simulink model "Target_Control_System"  (R2021b)
settings: Solver=FixedStepDiscrete  StartTime=0.0  StopTime=5  RelTol=1e-3
PreLoadFcn:
  | RTWConfigurationCB('preloadfcn', bdroot);
PostLoadFcn:
  | load('configuration/data_struct.mat');
  | load('configuration/fluxMaps_propMotor.mat');
  | load('configuration/parameterInit_PROP.mat');
  | load('configuration/parameterInit_PUMP.mat');
  | load('configuration/parameterInit_PITCH.mat');
  | load('configuration/parameterInit_TILT.mat');
  | %load('configuration/base_workspace_signal_definition.mat');
  | %load('resolvedatastores_to_baseworkspace_for_faster_simulation.mat');
model workspace (MAT data in the model file):
  SIMULATION_OPTIONS : Simulink.Parameter (value not decoded)
  TARGET_CODE_GEN : Simulink.Parameter (value not decoded)
  TCS_SAMPLE_FREQ_HZ : Simulink.Parameter (value not decoded)
symbols that are objects in the model workspace (value not decoded): TARGET_CODE_GEN, TCS_SAMPLE_FREQ_HZ
undefined symbols (not defined in the file): A_DQ_REF_LPF_INIT__PITCH, A_DQ_REF_LPF_INIT__PROP, A_DQ_REF_LPF_INIT__PUMP, A_DQ_REF_LPF_INIT__TILT, A_OBSERVER_CONFIDENCE_INIT__PITCH, A_OBSERVER_CONFIDENCE_INIT__PROP, A_OBSERVER_CONFIDENCE_INIT__PUMP, A_OBSERVER_CONFIDENCE_INIT__TILT, ACTUATOR_MAX_ANGLE_TRIP__PITCH, ACTUATOR_MIN_ANGLE_TRIP__PITCH, ACTUATOR_POS_SENSOR_INV_DIRECTION__PITCH, ACTUATOR_POS_SENSOR_INV_DIRECTION__TILT, ACTUATOR_POS_SENSOR_OFFSET__PITCH, ACTUATOR_POS_SENSOR_OFFSET__TILT, ADC_scaler1_baseaddr_TILT, ADC_SCALER_FLOAT_TO_FIXPOINT_EXPANSION, ANGLE_ELEC_FROM_SENSOR_OFFSET_INIT__PITCH, ANGLE_ELEC_FROM_SENSOR_OFFSET_INIT__PROP, ANGLE_ELEC_FROM_SENSOR_OFFSET_INIT__PUMP, ANGLE_ELEC_FROM_SENSOR_OFFSET_INIT__TILT, AUTO_CLEAR_FAULTS_ENABLED__PITCH, AUTO_CLEAR_FAULTS_ENABLED__PROP, AUTO_CLEAR_FAULTS_ENABLED__PUMP, AUTO_CLEAR_FAULTS_ENABLED__TILT, AUTO_CLEAR_FAULTS_WAIT_TICKS__PITCH, AUTO_CLEAR_FAULTS_WAIT_TICKS__PROP, AUTO_CLEAR_FAULTS_WAIT_TICKS__PUMP, AUTO_CLEAR_FAULTS_WAIT_TICKS__TILT, AUTO_I_ZERO_IDLE_TICKS__PITCH, AUTO_I_ZERO_IDLE_TICKS__PROP, AUTO_I_ZERO_IDLE_TICKS__PUMP, AUTO_I_ZERO_IDLE_TICKS__TILT, AUTO_I_ZERO_OFFSET_IDC_THRESHOLD__PITCH, AUTO_I_ZERO_OFFSET_IDC_THRESHOLD__PROP, AUTO_I_ZERO_OFFSET_IDC_THRESHOLD__PUMP, AUTO_I_ZERO_OFFSET_IDC_THRESHOLD__TILT, AUTO_I_ZERO_OFFSET_IPH_THRESHOLD__PITCH, AUTO_I_ZERO_OFFSET_IPH_THRESHOLD__PROP, AUTO_I_ZERO_OFFSET_IPH_THRESHOLD__PUMP, AUTO_I_ZERO_OFFSET_IPH_THRESHOLD__TILT, AUTO_SENSORLESS_SWITCHOVER_DISABLE_OMEGA, AUTO_SENSORLESS_SWITCHOVER_ENABLE_OMEGA, AUTO_SENSORLESS_SWITCHOVER_MIN_CONFIDENCE, AUXILIARY_PROTECTION_UNIT_BASEADDR__TILT, blanking_max_error_omega_INIT_PITCH, blanking_max_error_omega_INIT_TILT, blanking_max_error_position_INIT_PITCH, blanking_max_error_position_INIT_TILT, BRUTE_START_I_Q_REF_RAMP_SPEED__PITCH, BRUTE_START_I_Q_REF_RAMP_SPEED__PROP, BRUTE_START_I_Q_REF_RAMP_SPEED__PUMP, BRUTE_START_I_Q_REF_RAMP_SPEED__TILT, CONTROL_LOOP_DT_INIT__PITCH, CONTROL_LOOP_DT_INIT__PROP, CONTROL_LOOP_DT_INIT__PUMP, CONTROL_LOOP_DT_INIT__TILT, CORRECTION_FILTER_SCALE__PITCH, CORRECTION_FILTER_SCALE__PROP, CORRECTION_FILTER_SCALE__PUMP, CORRECTION_FILTER_SCALE__TILT ... (+458)
libraries: simulink x178, Reusables_Lib x24
(part 5 of 47)

== system Target_Control_System/Target_Control_System/Simulation Controls/Simulation Data Store Initialization ==
  note: This function initializes all of the data store variables for simulation purposes. This mimics the parameter_init_prop.c and parameter_init_prop.h that are used for hardware execution.
      | If a variable is defined in parameter_init_prop.h, then it is included in the Model Workspace as a Simulink parameter.
  Constant76 : Constant  Value=0  SampleTime=-1
  Digital Clock : DigitalClock  SampleTime=-1
  Equal : RelationalOperator  Operator===  OutDataTypeStr=boolean  RndMeth=Simplest
  Function-Call Split{,1..6,8..9,17..27} (20 alike) : FunctionCallSplit  NumOutputPorts=2
  initializationFlowControl : Subsystem  TreatAsAtomicUnit=on
  initializeDataForPitch() : Subsystem  Priority=1  TreatAsAtomicUnit=on
  initializeDataForTilt() : Subsystem  Priority=1  TreatAsAtomicUnit=on
  initializeTiltAsMaster() : Subsystem
  parameter_init_prop : Subsystem  TreatAsAtomicUnit=on
  parameter_init_pump : Subsystem  TreatAsAtomicUnit=on
  setHardwareCurrentLimitTilt()1 : Subsystem  Commented=on  TreatAsAtomicUnit=on
  setPositionControlModeTilt() : Subsystem
  setTiltMotorSpecificParameters() : Subsystem
  setupIirFilters(&oTilt) : Subsystem
  setupIirFilters() : Subsystem
  setupObserver(&oTilt) : Subsystem  TreatAsAtomicUnit=on
  setupObserver() : Subsystem
  setupObserverForPosSensor(&oTilt) : Subsystem
  setupPwm(&oTilt) : Subsystem
  setupPwm() : Subsystem
  updateIqSetpointMax(&oTilt) : Subsystem
  updateIqSetpointMax() : Subsystem
  updateServoObserver(&oTilt) : Subsystem
  updateServoObserver() : Subsystem
  updateSoftCurrentLimitTilt()1 : Subsystem  Commented=on  TreatAsAtomicUnit=on
  wires:
  Function-Call Split21/2 -> Function-Call Split20/1
  Function-Call Split9/1 -> updateIqSetpointMax()/Trigger
  Function-Call Split27/2 -> Function-Call Split19/1
  Function-Call Split22/1 -> updateIqSetpointMax(&oTilt)/Trigger
  Function-Call Split23/1 -> initializeTiltAsMaster()/Trigger
  Function-Call Split20/2 -> updateSoftCurrentLimitTilt()1/Trigger
  Function-Call Split24/2 -> Function-Call Split25/1
  Function-Call Split26/1 -> updateServoObserver(&oTilt)/Trigger
  Function-Call Split23/2 -> Function-Call Split21/1
  Function-Call Split18/2 -> Function-Call Split24/1
  Function-Call Split24/1 -> setupPwm(&oTilt)/Trigger
  Function-Call Split2/2 -> Function-Call Split17/1
  Function-Call Split19/2 -> Function-Call Split22/1
  Function-Call Split21/1 -> setPositionControlModeTilt()/Trigger
  Function-Call Split17/1 -> initializeDataForTilt()/Trigger
  Function-Call Split17/2 -> Function-Call Split18/1
  Function-Call Split26/2 -> Function-Call Split27/1
  Function-Call Split25/1 -> setupObserver(&oTilt)/Trigger
  Function-Call Split18/1 -> setTiltMotorSpecificParameters()/Trigger
  Function-Call Split27/1 -> setupObserverForPosSensor(&oTilt)/Trigger
  Function-Call Split20/1 -> setHardwareCurrentLimitTilt()1/Trigger
  Function-Call Split25/2 -> Function-Call Split26/1
  Function-Call Split22/2 -> Function-Call Split23/1
  Function-Call Split19/1 -> setupIirFilters(&oTilt)/Trigger
  Function-Call Split1/1 -> parameter_init_pump/Trigger
  Function-Call Split5/1 -> updateServoObserver()/Trigger
  Function-Call Split3/1 -> setupPwm()/Trigger
  Function-Call Split6/1 -> setupIirFilters()/Trigger
  Function-Call Split4/2 -> Function-Call Split5/1
  Function-Call Split4/1 -> setupObserver()/Trigger
  Function-Call Split5/2 -> Function-Call Split6/1
  Function-Call Split8/2 -> Function-Call Split3/1
  Function-Call Split6/2 -> Function-Call Split9/1
  Function-Call Split8/1 -> initializeDataForPitch()/Trigger
  Function-Call Split3/2 -> Function-Call Split4/1
  Equal/1 -> initializationFlowControl/Trigger
  Function-Call Split1/2 -> Function-Call Split2/1
  initializationFlowControl/1(Out1) -> Function-Call Split/1
  Function-Call Split/1 -> parameter_init_prop/Trigger
  Function-Call Split/2 -> Function-Call Split1/1
  Function-Call Split2/1 -> Function-Call Split8/1
  Constant76/1 -> Equal/2
  Digital Clock/1 -> Equal/1

== system Target_Control_System/Target_Control_System/Simulation Controls/pitchMotor ==
  pitchMotor_simControls : Inport
  Apply Simulation Parameter Values : Subsystem  TreatAsAtomicUnit=on
  Apply Simulation Setpoints : Subsystem  TreatAsAtomicUnit=on
  Bus Selector : BusSelector  OutputSignals=uiEnable
  Bus Selector1 : BusSelector  OutputSignals=controlSelector
  Bus Selector2 : BusSelector  OutputSignals=currentSetpoint,speedSetpoint,positionSetpoint
  Bus Selector3 : BusSelector  OutputSignals=OneOverSensorPolePairs
  Detect Change : simulink/Logic and Bit Operations/Detect Change  vinit=0  OutDataTypeStr=boolean
  Detect Change1 : simulink/Logic and Bit Operations/Detect Change  vinit=0  OutDataTypeStr=boolean
  Drive Enable : Subsystem  TreatAsAtomicUnit=on
  Initialize controller : Subsystem  TreatAsAtomicUnit=on
  wires:
  Bus Selector2/3 -> Apply Simulation Setpoints/4(Position Setpoint for Simulation)  "<positionSetpoint>"
  Bus Selector2/1 -> Apply Simulation Setpoints/2(Current Setpoint for Simulation)  "<currentSetpoint>"
  Bus Selector2/2 -> Apply Simulation Setpoints/3(Speed Setpoint for Simulation)  "<speedSetpoint>"
  Bus Selector1/1 -> Initialize controller/1(controllerSelection), Apply Simulation Setpoints/1(controllerSelection), Detect Change1/1  "<controlSelector>"
  pitchMotor_simControls/1 -> Bus Selector/1, Bus Selector3/1, Bus Selector2/1, Bus Selector1/1
  Detect Change1/1 -> Initialize controller/Trigger  "change"
  Bus Selector3/1 -> Apply Simulation Parameter Values/1(OneOverSensorPolePairs)  "<OneOverSensorPolePairs>"
  Bus Selector/1 -> Detect Change/1, Drive Enable/1(pitchMotor_uiEnable)  "<uiEnable>"
  Detect Change/1 -> Drive Enable/Trigger  "change"

== system Target_Control_System/Target_Control_System/Simulation Controls/pitchMotor1 ==
  pitchMotor_fpgaFeedback : Inport
  Bus Selector : BusSelector  OutputSignals=oPitch:oMot_:oOut_:uiGateDriverStatus_,mdl_pitch_uiFlags,mdl_pitch_uiAPUFlags,oPitch:oMot_:oState_:opInputResolverData_:uiControlReadback_
  Data Store Write : DataStoreWrite  DataStoreName=oPitch  DataStoreElements=oPitch.oMot_.oState_.opInputResolverData_.uiControlReadback_  IndexOptions=Index vector (dialog)  Indices=1  OutputSizes=1
  Data Store Write1 : DataStoreWrite  DataStoreName=mdl_pitch_uiFlags  IndexOptions=Index vector (dialog)  Indices=1  OutputSizes=1
  Data Store Write2 : DataStoreWrite  DataStoreName=mdl_pitch_uiAPUFlags  IndexOptions=Index vector (dialog)  Indices=1  OutputSizes=1
  Data Store Write43 : DataStoreWrite  DataStoreName=oPitch  DataStoreElements=oPitch.oMot_.oOut_.uiGateDriverStatus_  IndexOptions=Index vector (dialog)  Indices=1  OutputSizes=1
  wires:
  Bus Selector/4 -> Data Store Write/1  "<oPitch:oMot_:oState_:opInputResolverData_:uiControlReadback_>"
  pitchMotor_fpgaFeedback/1 -> Bus Selector/1
  Bus Selector/2 -> Data Store Write1/1  "<mdl_pitch_uiFlags>"
  Bus Selector/3 -> Data Store Write2/1  "<mdl_pitch_uiAPUFlags>"
  Bus Selector/1 -> Data Store Write43/1  "<oPitch:oMot_:oOut_:uiGateDriverStatus_>"

== system Target_Control_System/Target_Control_System/Simulation Controls/propMotor ==
  propMotor_simControls : Inport
  Bus Selector : BusSelector  OutputSignals=uiEnable
  Detect Change : simulink/Logic and Bit Operations/Detect Change  vinit=0  OutDataTypeStr=boolean
  Drive Enable : Subsystem  TreatAsAtomicUnit=on
  wires:
  Bus Selector/1 -> Drive Enable/1(propMotor_uiEnable), Detect Change/1  "<uiEnable>"
  propMotor_simControls/1 -> Bus Selector/1
  Detect Change/1 -> Drive Enable/Trigger  "change"

== system Target_Control_System/Target_Control_System/Simulation Controls/pumpMotor ==
  pitchMotor_simControls : Inport
  Bus Selector : BusSelector  OutputSignals=uiEnable
  Detect Change : simulink/Logic and Bit Operations/Detect Change  vinit=0  OutDataTypeStr=boolean
  Drive Enable : Subsystem  TreatAsAtomicUnit=on
  wires:
  Bus Selector/1 -> Drive Enable/1(pumpMotor_uiEnable), Detect Change/1  "<uiEnable>"
  pitchMotor_simControls/1 -> Bus Selector/1  "pumpMotor_simControls"
  Detect Change/1 -> Drive Enable/Trigger  "change"

== system Target_Control_System/Target_Control_System/Simulation Controls/tiltMotor ==
  pitchMotor_simControls : Inport
  Apply Simulation Parameter Values : Subsystem  TreatAsAtomicUnit=on
  Apply Simulation Setpoints : Subsystem  TreatAsAtomicUnit=on
  Bus Selector : BusSelector  OutputSignals=uiEnable
  Bus Selector1 : BusSelector  OutputSignals=controlSelector
  Bus Selector2 : BusSelector  OutputSignals=currentSetpoint,speedSetpoint,positionSetpoint
  Bus Selector3 : BusSelector  OutputSignals=OneOverSensorPolePairs,TiltReadheadCompensationEnabled
  Detect Change : simulink/Logic and Bit Operations/Detect Change  vinit=0  OutDataTypeStr=boolean
  Detect Change1 : simulink/Logic and Bit Operations/Detect Change  vinit=0  OutDataTypeStr=boolean
  Drive Enable : Subsystem  TreatAsAtomicUnit=on
  Initialize controller : Subsystem  TreatAsAtomicUnit=on
  wires:
  Detect Change1/1 -> Initialize controller/Trigger  "change"
  Bus Selector2/2 -> Apply Simulation Setpoints/3(Speed Setpoint for Simulation)  "<speedSetpoint>"
  Bus Selector2/1 -> Apply Simulation Setpoints/2(Current Setpoint for Simulation)  "<currentSetpoint>"
  Bus Selector2/3 -> Apply Simulation Setpoints/4(Position Setpoint for Simulation)  "<positionSetpoint>"
  Bus Selector1/1 -> Initialize controller/1(controllerSelection), Apply Simulation Setpoints/1(controllerSelection), Detect Change1/1  "<controlSelector>"
  Bus Selector3/2 -> Apply Simulation Parameter Values/2(TiltReadheadCompensationEnabled)  "<TiltReadheadCompensationEnabled>"
  Bus Selector3/1 -> Apply Simulation Parameter Values/1(OneOverSensorPolePairs)  "<OneOverSensorPolePairs>"
  Bus Selector/1 -> Drive Enable/1(tiltMotor_uiEnable), Detect Change/1  "<uiEnable>"
  pitchMotor_simControls/1 -> Bus Selector/1, Bus Selector3/1, Bus Selector2/1, Bus Selector1/1  "tiltMotor_simControls"
  Detect Change/1 -> Drive Enable/Trigger  "change"

== system Target_Control_System/Target_Control_System/Simulation Controls/tiltMotor1 ==
  tiltMotor_fpgaFeedback : Inport
  Bus Selector : BusSelector  OutputSignals=oTilt:oMot_:oOut_:uiGateDriverStatus_,mdl_tilt_uiFlags,mdl_tilt_uiAPUFlags,oTilt:oMot_:oState_:opInputResolverData_:uiControlReadback_,mdl_tilt_uiInputSensorFlags,mdl_tilt_uiOutputSensorFlags
  Data Store Write : DataStoreWrite  DataStoreName=oTilt  DataStoreElements=oTilt.oMot_.oState_.opInputResolverData_.uiControlReadback_  IndexOptions=Index vector (dialog)  Indices=1  OutputSizes=1
  Data Store Write1 : DataStoreWrite  DataStoreName=mdl_tilt_uiFlags  IndexOptions=Index vector (dialog)  Indices=1  OutputSizes=1
  Data Store Write2 : DataStoreWrite  DataStoreName=mdl_tilt_uiAPUFlags  IndexOptions=Index vector (dialog)  Indices=1  OutputSizes=1
  Data Store Write3 : DataStoreWrite  DataStoreName=mdl_tilt_uiInputSensorFlags  IndexOptions=Index vector (dialog)  Indices=1  OutputSizes=1
  Data Store Write4 : DataStoreWrite  DataStoreName=mdl_tilt_uiOutputSensorFlags  IndexOptions=Index vector (dialog)  Indices=1  OutputSizes=1
  Data Store Write43 : DataStoreWrite  DataStoreName=oTilt  DataStoreElements=oTilt.oMot_.oOut_.uiGateDriverStatus_  IndexOptions=Index vector (dialog)  Indices=1  OutputSizes=1
  wires:
  Bus Selector/6 -> Data Store Write4/1  "<mdl_tilt_uiOutputSensorFlags>"
  Bus Selector/5 -> Data Store Write3/1  "<mdl_tilt_uiInputSensorFlags>"
  Bus Selector/4 -> Data Store Write/1  "<oTilt:oMot_:oState_:opInputResolverData_:uiControlReadback_>"
  tiltMotor_fpgaFeedback/1 -> Bus Selector/1
  Bus Selector/2 -> Data Store Write1/1  "<mdl_tilt_uiFlags>"
  Bus Selector/3 -> Data Store Write2/1  "<mdl_tilt_uiAPUFlags>"
  Bus Selector/1 -> Data Store Write43/1  "<oTilt:oMot_:oOut_:uiGateDriverStatus_>"

== system Target_Control_System/Target_Control_System/DEBUG_Scopes/Pump Motor Debug/2Pi_Mod1 ==
  Iabc1 : Inport
  Constant : Constant  Value=pi  OutDataTypeStr=single  SampleTime=-1
  "Constant " : Constant  Value=pi  OutDataTypeStr=single  SampleTime=-1
  Math Function : Math  Operator=mod  SignedPower=on  SaturateOnIntegerOverflow=on
  Modulo Constant : Constant  Value=2*pi  OutDataTypeStr=single  SampleTime=-1
  Sum1 : Sum  Inputs=|++
  Sum2 : Sum  Inputs=|+-
  Out1 : Outport
  wires:
  Sum2/1 -> Out1/1
  Constant/1 -> Sum2/2
  Math Function/1 -> Sum2/1
  Sum1/1 -> Math Function/1
  Iabc1/1 -> Sum1/1
  "Constant "/1 -> Sum1/2
  Modulo Constant/1 -> Math Function/2

== system Target_Control_System/Target_Control_System/DEBUG_Scopes/Pump Motor Debug/2Pi_Mod2 ==
  Iabc1 : Inport
  Discrete Integrator Samples1 : Constant  Value=270/360*2*pi  OutDataTypeStr=single  SampleTime=-1
  Discrete Integrator Samples2 : Constant  Value=pi  OutDataTypeStr=single  SampleTime=-1
  Math Function : Math  Operator=mod  SignedPower=on  SaturateOnIntegerOverflow=on
  Modulo Constant : Constant  Value=2*pi  OutDataTypeStr=single  SampleTime=-1
  Sum1 : Sum  Inputs=|++
  Sum2 : Sum  Inputs=|+-
  Out1 : Outport
  wires:
  Sum2/1 -> Out1/1
  Discrete Integrator Samples2/1 -> Sum2/2
  Math Function/1 -> Sum2/1
  Sum1/1 -> Math Function/1
  Iabc1/1 -> Sum1/1
  Discrete Integrator Samples1/1 -> Sum1/2
  Modulo Constant/1 -> Math Function/2

== system Target_Control_System/Target_Control_System/DEBUG_Scopes/Pump Motor Debug/IIR3 ==
  Input : Inport
  Constant : Constant  Value=CoefficientA  OutDataTypeStr=single  SampleTime=-1
  Constant1 : Constant  Value=CoefficientB  OutDataTypeStr=single  SampleTime=-1
  Product : Product  OutDataTypeStr=single  RndMeth=Zero
  Product1 : Product  RndMeth=Zero
  Sum : Sum  Inputs=|++  OutDataTypeStr=single
  Unit Delay : UnitDelay  SampleTime=-1  HasFrameUpgradeWarning=on
  Output : Outport
  wires:
  Sum/1 -> Unit Delay/1, Output/1
  Unit Delay/1 -> Product/1
  Constant1/1 -> Product1/2
  Constant/1 -> Product/2
  Product/1 -> Sum/1
  Product1/1 -> Sum/2
  Input/1 -> Product1/1

== system Target_Control_System/Target_Control_System/DEBUG_Scopes/Pump Motor Debug/IIR4 ==
  Input : Inport
  Constant : Constant  Value=CoefficientA  OutDataTypeStr=single  SampleTime=-1
  Constant1 : Constant  Value=CoefficientB  OutDataTypeStr=single  SampleTime=-1
  Product : Product  OutDataTypeStr=single  RndMeth=Zero
  Product1 : Product  RndMeth=Zero
  Sum : Sum  Inputs=|++  OutDataTypeStr=single
  Unit Delay : UnitDelay  SampleTime=-1  HasFrameUpgradeWarning=on
  Output : Outport
  wires:
  Sum/1 -> Unit Delay/1, Output/1
  Unit Delay/1 -> Product/1
  Constant1/1 -> Product1/2
  Constant/1 -> Product/2
  Product/1 -> Sum/1
  Product1/1 -> Sum/2
  Input/1 -> Product1/1

== system Target_Control_System/Target_Control_System/InterruptFunction/allMotors_readAdc/codeGen_adcRead ==
  Enable : EnablePort
  Data Store Read24 : DataStoreRead  DataStoreName=oProp  DataStoreElements=oProp.oIsr_.oIn_.oAdcData_.fUa_  IndexOptions=Index vector (dialog)  Indices=1  OutputSizes=1
  Data Store Read25 : DataStoreRead  DataStoreName=oProp  DataStoreElements=oProp.oIsr_.oIn_.oAdcData_.fUb_  IndexOptions=Index vector (dialog)  Indices=1  OutputSizes=1
  Data Store Read26 : DataStoreRead  DataStoreName=oProp  DataStoreElements=oProp.oIsr_.oIn_.oAdcData_.fUc_  IndexOptions=Index vector (dialog)  Indices=1  OutputSizes=1
  Data Store Read27 : DataStoreRead  DataStoreName=oPitch  DataStoreElements=oPitch.oIsr_.oIn_.oAdcData_.fUa_  IndexOptions=Index vector (dialog)  Indices=1  OutputSizes=1
  Data Store Read30 : DataStoreRead  DataStoreName=oPitch  DataStoreElements=oPitch.oIsr_.oIn_.oAdcData_.fUb_  IndexOptions=Index vector (dialog)  Indices=1  OutputSizes=1
  Data Store Read33 : DataStoreRead  DataStoreName=oPump  DataStoreElements=oPump.oIsr_.oIn_.oAdcData_.fUa_  IndexOptions=Index vector (dialog)  Indices=1  OutputSizes=1
  Data Store Read34 : DataStoreRead  DataStoreName=oPump  DataStoreElements=oPump.oIsr_.oIn_.oAdcData_.fUb_  IndexOptions=Index vector (dialog)  Indices=1  OutputSizes=1
  Data Store Read35 : DataStoreRead  DataStoreName=oPump  DataStoreElements=oPump.oIsr_.oIn_.oAdcData_.fUc_  IndexOptions=Index vector (dialog)  Indices=1  OutputSizes=1
  Data Store Read36 : DataStoreRead  DataStoreName=oPitch  DataStoreElements=oPitch.oIsr_.oIn_.oAdcData_.fUc_  IndexOptions=Index vector (dialog)  Indices=1  OutputSizes=1
  Data Store Read39 : DataStoreRead  DataStoreName=oTilt  DataStoreElements=oTilt.oIsr_.oIn_.oAdcData_.fUa_  IndexOptions=Index vector (dialog)  Indices=1  OutputSizes=1
  Data Store Read4 : DataStoreRead  DataStoreName=oPump  DataStoreElements=oPump.oIsr_.oIn_.oAdcData_.fUdc_  IndexOptions=Index vector (dialog)  Indices=1  OutputSizes=1
  Data Store Read41 : DataStoreRead  DataStoreName=oTilt  DataStoreElements=oTilt.oIsr_.oIn_.oAdcData_.fUb_  IndexOptions=Index vector (dialog)  Indices=1  OutputSizes=1
  Data Store Read42 : DataStoreRead  DataStoreName=oTilt  DataStoreElements=oTilt.oIsr_.oIn_.oAdcData_.fUc_  IndexOptions=Index vector (dialog)  Indices=1  OutputSizes=1
  Data Store Read8 : DataStoreRead  DataStoreName=oProp  DataStoreElements=oProp.oIsr_.oIn_.oAdcData_.fUdc_  IndexOptions=Index vector (dialog)  Indices=1  OutputSizes=1
  Data Store Write10 : DataStoreWrite  DataStoreName=oTilt  DataStoreElements=oTilt.oIsr_.oState_.fUdcPostlpf_  IndexOptions=Index vector (dialog)  Indices=1  OutputSizes=1
  Data Store Write11 : DataStoreWrite  DataStoreName=oProp  DataStoreElements=oProp.oIsr_.oState_.fUaPostlpf_  IndexOptions=Index vector (dialog)  Indices=1  OutputSizes=1
  Data Store Write12 : DataStoreWrite  DataStoreName=oProp  DataStoreElements=oProp.oIsr_.oState_.fUbPostlpf_  IndexOptions=Index vector (dialog)  Indices=1  OutputSizes=1
  Data Store Write13 : DataStoreWrite  DataStoreName=oProp  DataStoreElements=oProp.oIsr_.oState_.fUcPostlpf_  IndexOptions=Index vector (dialog)  Indices=1  OutputSizes=1
  Data Store Write22 : DataStoreWrite  DataStoreName=oPump  DataStoreElements=oPump.oIsr_.oState_.fUaPostlpf_  IndexOptions=Index vector (dialog)  Indices=1  OutputSizes=1
  Data Store Write23 : DataStoreWrite  DataStoreName=oPump  DataStoreElements=oPump.oIsr_.oState_.fUbPostlpf_  IndexOptions=Index vector (dialog)  Indices=1  OutputSizes=1
  Data Store Write24 : DataStoreWrite  DataStoreName=oPump  DataStoreElements=oPump.oIsr_.oState_.fUcPostlpf_  IndexOptions=Index vector (dialog)  Indices=1  OutputSizes=1
  Data Store Write3 : DataStoreWrite  DataStoreName=oPitch  DataStoreElements=oPitch.oIsr_.oIn_.oAdcData_.fUdc_  IndexOptions=Index vector (dialog)  Indices=1  OutputSizes=1
  Data Store Write31 : DataStoreWrite  DataStoreName=oPitch  DataStoreElements=oPitch.oIsr_.oState_.fUaPostlpf_  IndexOptions=Index vector (dialog)  Indices=1  OutputSizes=1
  Data Store Write32 : DataStoreWrite  DataStoreName=oPitch  DataStoreElements=oPitch.oIsr_.oState_.fUbPostlpf_  IndexOptions=Index vector (dialog)  Indices=1  OutputSizes=1
  Data Store Write33 : DataStoreWrite  DataStoreName=oPitch  DataStoreElements=oPitch.oIsr_.oState_.fUcPostlpf_  IndexOptions=Index vector (dialog)  Indices=1  OutputSizes=1
  Data Store Write37 : DataStoreWrite  DataStoreName=oTilt  DataStoreElements=oTilt.oIsr_.oState_.fUaPostlpf_  IndexOptions=Index vector (dialog)  Indices=1  OutputSizes=1
  Data Store Write38 : DataStoreWrite  DataStoreName=oTilt  DataStoreElements=oTilt.oIsr_.oState_.fUbPostlpf_  IndexOptions=Index vector (dialog)  Indices=1  OutputSizes=1
  Data Store Write39 : DataStoreWrite  DataStoreName=oTilt  DataStoreElements=oTilt.oIsr_.oState_.fUcPostlpf_  IndexOptions=Index vector (dialog)  Indices=1  OutputSizes=1
  Data Store Write4 : DataStoreWrite  DataStoreName=oPump  DataStoreElements=oPump.oIsr_.oState_.fUdcPostlpf_  IndexOptions=Index vector (dialog)  Indices=1  OutputSizes=1
  Data Store Write5 : DataStoreWrite  DataStoreName=oProp  DataStoreElements=oProp.oIsr_.oState_.fUdcPostlpf_  IndexOptions=Index vector (dialog)  Indices=1  OutputSizes=1
  Data Store Write6 : DataStoreWrite  DataStoreName=oTilt  DataStoreElements=oTilt.oIsr_.oIn_.oAdcData_.fUdc_  IndexOptions=Index vector (dialog)  Indices=1  OutputSizes=1
  Data Store Write7 : DataStoreWrite  DataStoreName=oPitch  DataStoreElements=oPitch.oIsr_.oState_.fUdcPostlpf_  IndexOptions=Index vector (dialog)  Indices=1  OutputSizes=1
  wires:
  Data Store Read8/1 -> Data Store Write5/1  "Udc"
  Data Store Read4/1 -> Data Store Write4/1, Data Store Write3/1, Data Store Write7/1, Data Store Write6/1, Data Store Write10/1  "Ua"
  Data Store Read39/1 -> Data Store Write37/1
  Data Store Read41/1 -> Data Store Write38/1
  Data Store Read27/1 -> Data Store Write31/1
  Data Store Read25/1 -> Data Store Write12/1
  Data Store Read42/1 -> Data Store Write39/1
  Data Store Read24/1 -> Data Store Write11/1
  Data Store Read34/1 -> Data Store Write23/1
  Data Store Read30/1 -> Data Store Write32/1
  Data Store Read35/1 -> Data Store Write24/1
  Data Store Read33/1 -> Data Store Write22/1
  Data Store Read26/1 -> Data Store Write13/1
  Data Store Read36/1 -> Data Store Write33/1

== system Target_Control_System/Target_Control_System/InterruptFunction/allMotors_readAdc/pitchMotor_adcRead ==
  PitchMotorAdcFeedback : Inport  OutDataTypeStr=Bus: SAdcDataSingleIn_t  PortDimensions=[ 1 ]  BusOutputAsStruct=on
  Enable : EnablePort
  Bus Selector : BusSelector  OutputSignals=fIa_,fIb_,fIc_,fIdc_,fUa_,fUb_,fUc_,fUdc_,fAuxiliaryEncoderFloat_,fMotorEncoderFloat_,fMotorSensorSpeed_,fOutputEncoderFloat_,fOutputSensorSpeed_
  Data Store Write : DataStoreWrite  DataStoreName=oPitch  DataStoreElements=oPitch.oIsr_.oIn_.oAdcData_.fIa_  IndexOptions=Index vector (dialog)  Indices=1  OutputSizes=1
  Data Store Write1 : DataStoreWrite  DataStoreName=oPitch  DataStoreElements=oPitch.oIsr_.oIn_.oAdcData_.fIb_  IndexOptions=Index vector (dialog)  Indices=1  OutputSizes=1
  Data Store Write10 : DataStoreWrite  DataStoreName=oPitch  DataStoreElements=oPitch.oIsr_.oIn_.oAdcData_.fMotorSensorSpeed_  IndexOptions=Index vector (dialog)  Indices=1  OutputSizes=1
  Data Store Write11 : DataStoreWrite  DataStoreName=oPitch  DataStoreElements=oPitch.oIsr_.oIn_.oAdcData_.fOutputEncoderFloat_  IndexOptions=Index vector (dialog)  Indices=1  OutputSizes=1
  Data Store Write12 : DataStoreWrite  DataStoreName=oPitch  DataStoreElements=oPitch.oIsr_.oIn_.oAdcData_.fOutputSensorSpeed_  IndexOptions=Index vector (dialog)  Indices=1  OutputSizes=1
  Data Store Write13 : DataStoreWrite  DataStoreName=oPitch  DataStoreElements=oPitch.oIsr_.oOut_.fUdc_  IndexOptions=Index vector (dialog)  Indices=1  OutputSizes=1
  Data Store Write14 : DataStoreWrite  DataStoreName=oPitch  DataStoreElements=oPitch.oIsr_.oState_.fUaPostlpf_  IndexOptions=Index vector (dialog)  Indices=1  OutputSizes=1
  Data Store Write15 : DataStoreWrite  DataStoreName=oPitch  DataStoreElements=oPitch.oIsr_.oState_.fUbPostlpf_  IndexOptions=Index vector (dialog)  Indices=1  OutputSizes=1
  Data Store Write16 : DataStoreWrite  DataStoreName=oPitch  DataStoreElements=oPitch.oIsr_.oState_.fUcPostlpf_  IndexOptions=Index vector (dialog)  Indices=1  OutputSizes=1
  Data Store Write19 : DataStoreWrite  DataStoreName=oPitch  DataStoreElements=oPitch.oIsr_.oState_.fUdcPostlpf_  IndexOptions=Index vector (dialog)  Indices=1  OutputSizes=1
  Data Store Write2 : DataStoreWrite  DataStoreName=oPitch  DataStoreElements=oPitch.oIsr_.oIn_.oAdcData_.fIc_  IndexOptions=Index vector (dialog)  Indices=1  OutputSizes=1
  Data Store Write3 : DataStoreWrite  DataStoreName=oPitch  DataStoreElements=oPitch.oIsr_.oIn_.oAdcData_.fIdc_  IndexOptions=Index vector (dialog)  Indices=1  OutputSizes=1
  Data Store Write4 : DataStoreWrite  DataStoreName=oPitch  DataStoreElements=oPitch.oIsr_.oIn_.oAdcData_.fUa_  IndexOptions=Index vector (dialog)  Indices=1  OutputSizes=1
  Data Store Write5 : DataStoreWrite  DataStoreName=oPitch  DataStoreElements=oPitch.oIsr_.oIn_.oAdcData_.fUb_  IndexOptions=Index vector (dialog)  Indices=1  OutputSizes=1
  Data Store Write6 : DataStoreWrite  DataStoreName=oPitch  DataStoreElements=oPitch.oIsr_.oIn_.oAdcData_.fUc_  IndexOptions=Index vector (dialog)  Indices=1  OutputSizes=1
  Data Store Write7 : DataStoreWrite  DataStoreName=oPitch  DataStoreElements=oPitch.oIsr_.oIn_.oAdcData_.fUdc_  IndexOptions=Index vector (dialog)  Indices=1  OutputSizes=1
  Data Store Write8 : DataStoreWrite  DataStoreName=oPitch  DataStoreElements=oPitch.oIsr_.oIn_.oAdcData_.fAuxiliaryEncoderFloat_  IndexOptions=Index vector (dialog)  Indices=1  OutputSizes=1
  Data Store Write9 : DataStoreWrite  DataStoreName=oPitch  DataStoreElements=oPitch.oIsr_.oIn_.oAdcData_.fMotorEncoderFloat_  IndexOptions=Index vector (dialog)  Indices=1  OutputSizes=1
  wires:
  Bus Selector/13 -> Data Store Write12/1  "<fOutputSensorSpeed_>"
  Bus Selector/2 -> Data Store Write1/1  "<fIb_>"
  Bus Selector/1 -> Data Store Write/1  "<fIa_>"
  Bus Selector/5 -> Data Store Write4/1, Data Store Write14/1  "<fUa_>"
  Bus Selector/8 -> Data Store Write19/1, Data Store Write13/1, Data Store Write7/1  "<fUdc_>"
  Bus Selector/9 -> Data Store Write8/1  "<fAuxiliaryEncoderFloat_>"
  Bus Selector/3 -> Data Store Write2/1  "<fIc_>"
  PitchMotorAdcFeedback/1 -> Bus Selector/1
  Bus Selector/6 -> Data Store Write5/1, Data Store Write15/1  "<fUb_>"
  Bus Selector/12 -> Data Store Write11/1  "<fOutputEncoderFloat_>"
  Bus Selector/11 -> Data Store Write10/1  "<fMotorSensorSpeed_>"
  Bus Selector/4 -> Data Store Write3/1  "<fIdc_>"
  Bus Selector/10 -> Data Store Write9/1  "<fMotorEncoderFloat_>"
  Bus Selector/7 -> Data Store Write6/1, Data Store Write16/1  "<fUc_>"

== system Target_Control_System/Target_Control_System/InterruptFunction/allMotors_readAdc/powerCalculations ==
  Data Store Read1 : DataStoreRead  DataStoreName=oPitch  DataStoreElements=oPitch.oIsr_.oIn_.oAdcData_.fIdc_  IndexOptions=Index vector (dialog)  Indices=1  OutputSizes=1
  Data Store Read10 : DataStoreRead  DataStoreName=oPitch  DataStoreElements=oPitch.oIsr_.oState_.fUdcPostlpf_  IndexOptions=Index vector (dialog)  Indices=1  OutputSizes=1
  Data Store Read11 : DataStoreRead  DataStoreName=oProp  DataStoreElements=oProp.oIsr_.oState_.fUdcPostlpf_  IndexOptions=Index vector (dialog)  Indices=1  OutputSizes=1
  Data Store Read12 : DataStoreRead  DataStoreName=oPitch  DataStoreElements=oPitch.oIsr_.oState_.fUdcPostlpf_  IndexOptions=Index vector (dialog)  Indices=1  OutputSizes=1
  Data Store Read15 : DataStoreRead  DataStoreName=oPump  DataStoreElements=oPump.oIsr_.oState_.fUdcPostlpf_  IndexOptions=Index vector (dialog)  Indices=1  OutputSizes=1
  Data Store Read16 : DataStoreRead  DataStoreName=oTilt  DataStoreElements=oTilt.oIsr_.oIn_.oAdcData_.fIdc_  IndexOptions=Index vector (dialog)  Indices=1  OutputSizes=1
  Data Store Read17 : DataStoreRead  DataStoreName=oTilt  DataStoreElements=oTilt.oIsr_.oState_.fUdcPostlpf_  IndexOptions=Index vector (dialog)  Indices=1  OutputSizes=1
  Data Store Read18 : DataStoreRead  DataStoreName=oTilt  DataStoreElements=oTilt.oIsr_.oState_.fUdcPostlpf_  IndexOptions=Index vector (dialog)  Indices=1  OutputSizes=1
  Data Store Read3 : DataStoreRead  DataStoreName=oProp  DataStoreElements=oProp.oIsr_.oState_.fUdcPostlpf_  IndexOptions=Index vector (dialog)  Indices=1  OutputSizes=1
  Data Store Read53 : DataStoreRead  DataStoreName=oProp  DataStoreElements=oProp.oIsr_.oIn_.oAdcData_.fIdc_  IndexOptions=Index vector (dialog)  Indices=1  OutputSizes=1
  Data Store Read6 : DataStoreRead  DataStoreName=oPump  DataStoreElements=oPump.oIsr_.oState_.fUdcPostlpf_  IndexOptions=Index vector (dialog)  Indices=1  OutputSizes=1
  Data Store Read9 : DataStoreRead  DataStoreName=oPump  DataStoreElements=oPump.oIsr_.oIn_.oAdcData_.fIdc_  IndexOptions=Index vector (dialog)  Indices=1  OutputSizes=1
  Data Store Write1 : DataStoreWrite  DataStoreName=oPitch  DataStoreElements=oPitch.oIsr_.oOut_.fPowerDc_  IndexOptions=Index vector (dialog)  Indices=1  OutputSizes=1
  Data Store Write14 : DataStoreWrite  DataStoreName=oProp  DataStoreElements=oProp.oIsr_.oOut_.fUdc_  IndexOptions=Index vector (dialog)  Indices=1  OutputSizes=1
  Data Store Write15 : DataStoreWrite  DataStoreName=oPump  DataStoreElements=oPump.oIsr_.oOut_.fPowerDc_  IndexOptions=Index vector (dialog)  Indices=1  OutputSizes=1
  Data Store Write19 : DataStoreWrite  DataStoreName=oTilt  DataStoreElements=oTilt.oIsr_.oOut_.fPowerDc_  IndexOptions=Index vector (dialog)  Indices=1  OutputSizes=1
  Data Store Write42 : DataStoreWrite  DataStoreName=oTilt  DataStoreElements=oTilt.oIsr_.oOut_.fUdc_  IndexOptions=Index vector (dialog)  Indices=1  OutputSizes=1
  Data Store Write5 : DataStoreWrite  DataStoreName=oPitch  DataStoreElements=oPitch.oIsr_.oOut_.fUdc_  IndexOptions=Index vector (dialog)  Indices=1  OutputSizes=1
  Data Store Write8 : DataStoreWrite  DataStoreName=oProp  DataStoreElements=oProp.oIsr_.oOut_.fPowerDc_  IndexOptions=Index vector (dialog)  Indices=1  OutputSizes=1
  Data Store Write9 : DataStoreWrite  DataStoreName=oPump  DataStoreElements=oPump.oIsr_.oOut_.fUdc_  IndexOptions=Index vector (dialog)  Indices=1  OutputSizes=1
  Product{1..3,11} (4 alike) : Product
  wires:
  Data Store Read18/1 -> Data Store Write42/1
  Data Store Read15/1 -> Data Store Write9/1
  Data Store Read11/1 -> Data Store Write14/1
  Data Store Read12/1 -> Data Store Write5/1
  Data Store Read17/1 -> Product3/1
  Product3/1 -> Data Store Write19/1
  Data Store Read16/1 -> Product3/2
  Data Store Read10/1 -> Product2/1
  Data Store Read3/1 -> Product11/1
  Data Store Read1/1 -> Product2/2
  Product1/1 -> Data Store Write15/1
  Data Store Read53/1 -> Product11/2
  Data Store Read6/1 -> Product1/1
  Product11/1 -> Data Store Write8/1
  Product2/1 -> Data Store Write1/1
  Data Store Read9/1 -> Product1/2

== system Target_Control_System/Target_Control_System/InterruptFunction/allMotors_readAdc/propMotor_adcRead ==
  PropMotorAdcFeedback : Inport  OutDataTypeStr=Bus: SAdcDataSingleIn_t  PortDimensions=[ 1 ]  BusOutputAsStruct=on
  Enable : EnablePort
  Bus Selector : BusSelector  OutputSignals=fIa_,fIb_,fIc_,fIdc_,fUa_,fUb_,fUc_,fUdc_,fAuxiliaryEncoderFloat_,fMotorEncoderFloat_,fMotorSensorSpeed_,fOutputEncoderFloat_,fOutputSensorSpeed_
  Data Store Write : DataStoreWrite  DataStoreName=oProp  DataStoreElements=oProp.oIsr_.oIn_.oAdcData_.fIa_  IndexOptions=Index vector (dialog)  Indices=1  OutputSizes=1
  Data Store Write1 : DataStoreWrite  DataStoreName=oProp  DataStoreElements=oProp.oIsr_.oIn_.oAdcData_.fIb_  IndexOptions=Index vector (dialog)  Indices=1  OutputSizes=1
  Data Store Write10 : DataStoreWrite  DataStoreName=oProp  DataStoreElements=oProp.oIsr_.oIn_.oAdcData_.fMotorSensorSpeed_  IndexOptions=Index vector (dialog)  Indices=1  OutputSizes=1
  Data Store Write11 : DataStoreWrite  DataStoreName=oProp  DataStoreElements=oProp.oIsr_.oIn_.oAdcData_.fOutputEncoderFloat_  IndexOptions=Index vector (dialog)  Indices=1  OutputSizes=1
  Data Store Write12 : DataStoreWrite  DataStoreName=oProp  DataStoreElements=oProp.oIsr_.oIn_.oAdcData_.fOutputSensorSpeed_  IndexOptions=Index vector (dialog)  Indices=1  OutputSizes=1
  Data Store Write13 : DataStoreWrite  DataStoreName=oProp  DataStoreElements=oProp.oIsr_.oOut_.fUdc_  IndexOptions=Index vector (dialog)  Indices=1  OutputSizes=1
  Data Store Write14 : DataStoreWrite  DataStoreName=oProp  DataStoreElements=oProp.oIsr_.oState_.fUaPostlpf_  IndexOptions=Index vector (dialog)  Indices=1  OutputSizes=1
  Data Store Write15 : DataStoreWrite  DataStoreName=oProp  DataStoreElements=oProp.oIsr_.oState_.fUbPostlpf_  IndexOptions=Index vector (dialog)  Indices=1  OutputSizes=1
  Data Store Write16 : DataStoreWrite  DataStoreName=oProp  DataStoreElements=oProp.oIsr_.oState_.fUcPostlpf_  IndexOptions=Index vector (dialog)  Indices=1  OutputSizes=1
  Data Store Write19 : DataStoreWrite  DataStoreName=oProp  DataStoreElements=oProp.oIsr_.oState_.fUdcPostlpf_  IndexOptions=Index vector (dialog)  Indices=1  OutputSizes=1
  Data Store Write2 : DataStoreWrite  DataStoreName=oProp  DataStoreElements=oProp.oIsr_.oIn_.oAdcData_.fIc_  IndexOptions=Index vector (dialog)  Indices=1  OutputSizes=1
  Data Store Write3 : DataStoreWrite  DataStoreName=oProp  DataStoreElements=oProp.oIsr_.oIn_.oAdcData_.fIdc_  IndexOptions=Index vector (dialog)  Indices=1  OutputSizes=1
  Data Store Write4 : DataStoreWrite  DataStoreName=oProp  DataStoreElements=oProp.oIsr_.oIn_.oAdcData_.fUa_  IndexOptions=Index vector (dialog)  Indices=1  OutputSizes=1
  Data Store Write5 : DataStoreWrite  DataStoreName=oProp  DataStoreElements=oProp.oIsr_.oIn_.oAdcData_.fUb_  IndexOptions=Index vector (dialog)  Indices=1  OutputSizes=1
  Data Store Write6 : DataStoreWrite  DataStoreName=oProp  DataStoreElements=oProp.oIsr_.oIn_.oAdcData_.fUc_  IndexOptions=Index vector (dialog)  Indices=1  OutputSizes=1
  Data Store Write7 : DataStoreWrite  DataStoreName=oProp  DataStoreElements=oProp.oIsr_.oIn_.oAdcData_.fUdc_  IndexOptions=Index vector (dialog)  Indices=1  OutputSizes=1
  Data Store Write8 : DataStoreWrite  DataStoreName=oProp  DataStoreElements=oProp.oIsr_.oIn_.oAdcData_.fAuxiliaryEncoderFloat_  IndexOptions=Index vector (dialog)  Indices=1  OutputSizes=1
  Data Store Write9 : DataStoreWrite  DataStoreName=oProp  DataStoreElements=oProp.oIsr_.oIn_.oAdcData_.fMotorEncoderFloat_  IndexOptions=Index vector (dialog)  Indices=1  OutputSizes=1
  wires:
  PropMotorAdcFeedback/1 -> Bus Selector/1
  Bus Selector/9 -> Data Store Write8/1  "<fAuxiliaryEncoderFloat_>"
  Bus Selector/10 -> Data Store Write9/1  "<fMotorEncoderFloat_>"
  Bus Selector/8 -> Data Store Write7/1, Data Store Write13/1, Data Store Write19/1  "<fUdc_>"
  Bus Selector/3 -> Data Store Write2/1  "<fIc_>"
  Bus Selector/2 -> Data Store Write1/1  "<fIb_>"
  Bus Selector/7 -> Data Store Write6/1, Data Store Write16/1  "<fUc_>"
  Bus Selector/11 -> Data Store Write10/1  "<fMotorSensorSpeed_>"
  Bus Selector/5 -> Data Store Write4/1, Data Store Write14/1  "<fUa_>"
  Bus Selector/4 -> Data Store Write3/1  "<fIdc_>"
  Bus Selector/12 -> Data Store Write11/1  "<fOutputEncoderFloat_>"
  Bus Selector/13 -> Data Store Write12/1  "<fOutputSensorSpeed_>"
  Bus Selector/1 -> Data Store Write/1  "<fIa_>"
  Bus Selector/6 -> Data Store Write5/1, Data Store Write15/1  "<fUb_>"

== system Target_Control_System/Target_Control_System/InterruptFunction/allMotors_readAdc/pumpMotor_adcRead ==
  PumpMotorAdcFeedback : Inport  OutDataTypeStr=Bus: SAdcDataSingleIn_t  PortDimensions=[ 1 ]  BusOutputAsStruct=on
  Enable : EnablePort
  Bus Selector : BusSelector  OutputSignals=fIa_,fIb_,fIc_,fIdc_,fUa_,fUb_,fUc_,fUdc_,fAuxiliaryEncoderFloat_,fMotorEncoderFloat_,fMotorSensorSpeed_,fOutputEncoderFloat_,fOutputSensorSpeed_
  Data Store Write : DataStoreWrite  DataStoreName=oPump  DataStoreElements=oPump.oIsr_.oIn_.oAdcData_.fIa_  IndexOptions=Index vector (dialog)  Indices=1  OutputSizes=1
  Data Store Write1 : DataStoreWrite  DataStoreName=oPump  DataStoreElements=oPump.oIsr_.oIn_.oAdcData_.fIb_  IndexOptions=Index vector (dialog)  Indices=1  OutputSizes=1
  Data Store Write10 : DataStoreWrite  DataStoreName=oPump  DataStoreElements=oPump.oIsr_.oIn_.oAdcData_.fMotorSensorSpeed_  IndexOptions=Index vector (dialog)  Indices=1  OutputSizes=1
  Data Store Write11 : DataStoreWrite  DataStoreName=oPump  DataStoreElements=oPump.oIsr_.oIn_.oAdcData_.fOutputEncoderFloat_  IndexOptions=Index vector (dialog)  Indices=1  OutputSizes=1
  Data Store Write12 : DataStoreWrite  DataStoreName=oPump  DataStoreElements=oPump.oIsr_.oIn_.oAdcData_.fOutputSensorSpeed_  IndexOptions=Index vector (dialog)  Indices=1  OutputSizes=1
  Data Store Write13 : DataStoreWrite  DataStoreName=oPump  DataStoreElements=oPump.oIsr_.oOut_.fUdc_  IndexOptions=Index vector (dialog)  Indices=1  OutputSizes=1
  Data Store Write14 : DataStoreWrite  DataStoreName=oPump  DataStoreElements=oPump.oIsr_.oState_.fUaPostlpf_  IndexOptions=Index vector (dialog)  Indices=1  OutputSizes=1
  Data Store Write15 : DataStoreWrite  DataStoreName=oPump  DataStoreElements=oPump.oIsr_.oState_.fUbPostlpf_  IndexOptions=Index vector (dialog)  Indices=1  OutputSizes=1
  Data Store Write16 : DataStoreWrite  DataStoreName=oPump  DataStoreElements=oPump.oIsr_.oState_.fUcPostlpf_  IndexOptions=Index vector (dialog)  Indices=1  OutputSizes=1
  Data Store Write19 : DataStoreWrite  DataStoreName=oPump  DataStoreElements=oPump.oIsr_.oState_.fUdcPostlpf_  IndexOptions=Index vector (dialog)  Indices=1  OutputSizes=1
  Data Store Write2 : DataStoreWrite  DataStoreName=oPump  DataStoreElements=oPump.oIsr_.oIn_.oAdcData_.fIc_  IndexOptions=Index vector (dialog)  Indices=1  OutputSizes=1
  Data Store Write3 : DataStoreWrite  DataStoreName=oPump  DataStoreElements=oPump.oIsr_.oIn_.oAdcData_.fIdc_  IndexOptions=Index vector (dialog)  Indices=1  OutputSizes=1
  Data Store Write4 : DataStoreWrite  DataStoreName=oPump  DataStoreElements=oPump.oIsr_.oIn_.oAdcData_.fUa_  IndexOptions=Index vector (dialog)  Indices=1  OutputSizes=1
  Data Store Write5 : DataStoreWrite  DataStoreName=oPump  DataStoreElements=oPump.oIsr_.oIn_.oAdcData_.fUb_  IndexOptions=Index vector (dialog)  Indices=1  OutputSizes=1
  Data Store Write6 : DataStoreWrite  DataStoreName=oPump  DataStoreElements=oPump.oIsr_.oIn_.oAdcData_.fUc_  IndexOptions=Index vector (dialog)  Indices=1  OutputSizes=1
  Data Store Write7 : DataStoreWrite  DataStoreName=oPump  DataStoreElements=oPump.oIsr_.oIn_.oAdcData_.fUdc_  IndexOptions=Index vector (dialog)  Indices=1  OutputSizes=1
  Data Store Write8 : DataStoreWrite  DataStoreName=oPump  DataStoreElements=oPump.oIsr_.oIn_.oAdcData_.fAuxiliaryEncoderFloat_  IndexOptions=Index vector (dialog)  Indices=1  OutputSizes=1
  Data Store Write9 : DataStoreWrite  DataStoreName=oPump  DataStoreElements=oPump.oIsr_.oIn_.oAdcData_.fMotorEncoderFloat_  IndexOptions=Index vector (dialog)  Indices=1  OutputSizes=1
  wires:
  Bus Selector/13 -> Data Store Write12/1  "<fOutputSensorSpeed_>"
  Bus Selector/2 -> Data Store Write1/1  "<fIb_>"
  Bus Selector/1 -> Data Store Write/1  "<fIa_>"
  Bus Selector/5 -> Data Store Write4/1, Data Store Write14/1  "<fUa_>"
  Bus Selector/8 -> Data Store Write19/1, Data Store Write13/1, Data Store Write7/1  "<fUdc_>"
  Bus Selector/9 -> Data Store Write8/1  "<fAuxiliaryEncoderFloat_>"
  Bus Selector/3 -> Data Store Write2/1  "<fIc_>"
  PumpMotorAdcFeedback/1 -> Bus Selector/1
  Bus Selector/6 -> Data Store Write5/1, Data Store Write15/1  "<fUb_>"
  Bus Selector/12 -> Data Store Write11/1  "<fOutputEncoderFloat_>"
  Bus Selector/11 -> Data Store Write10/1  "<fMotorSensorSpeed_>"
  Bus Selector/4 -> Data Store Write3/1  "<fIdc_>"
  Bus Selector/10 -> Data Store Write9/1  "<fMotorEncoderFloat_>"
  Bus Selector/7 -> Data Store Write6/1, Data Store Write16/1  "<fUc_>"

== system Target_Control_System/Target_Control_System/InterruptFunction/allMotors_readAdc/tiltMotor_adcRead ==
  TiltMotorAdcFeedback : Inport  OutDataTypeStr=Bus: SAdcDataSingleIn_t  PortDimensions=[ 1 ]  BusOutputAsStruct=on
  Enable : EnablePort
  Bus Selector : BusSelector  OutputSignals=fIa_,fIb_,fIc_,fIdc_,fUa_,fUb_,fUc_,fUdc_,fAuxiliaryEncoderFloat_,fMotorEncoderFloat_,fMotorSensorSpeed_,fOutputEncoderFloat_,fOutputSensorSpeed_
  Data Store Write : DataStoreWrite  DataStoreName=oTilt  DataStoreElements=oTilt.oIsr_.oIn_.oAdcData_.fIa_  IndexOptions=Index vector (dialog)  Indices=1  OutputSizes=1
  Data Store Write1 : DataStoreWrite  DataStoreName=oTilt  DataStoreElements=oTilt.oIsr_.oIn_.oAdcData_.fIb_  IndexOptions=Index vector (dialog)  Indices=1  OutputSizes=1
  Data Store Write10 : DataStoreWrite  DataStoreName=oTilt  DataStoreElements=oTilt.oIsr_.oIn_.oAdcData_.fMotorSensorSpeed_  IndexOptions=Index vector (dialog)  Indices=1  OutputSizes=1
  Data Store Write11 : DataStoreWrite  DataStoreName=oTilt  DataStoreElements=oTilt.oIsr_.oIn_.oAdcData_.fOutputEncoderFloat_  IndexOptions=Index vector (dialog)  Indices=1  OutputSizes=1
  Data Store Write12 : DataStoreWrite  DataStoreName=oTilt  DataStoreElements=oTilt.oIsr_.oIn_.oAdcData_.fOutputSensorSpeed_  IndexOptions=Index vector (dialog)  Indices=1  OutputSizes=1
  Data Store Write13 : DataStoreWrite  DataStoreName=oTilt  DataStoreElements=oTilt.oIsr_.oOut_.fUdc_  IndexOptions=Index vector (dialog)  Indices=1  OutputSizes=1
  Data Store Write14 : DataStoreWrite  DataStoreName=oTilt  DataStoreElements=oTilt.oIsr_.oState_.fUaPostlpf_  IndexOptions=Index vector (dialog)  Indices=1  OutputSizes=1
  Data Store Write15 : DataStoreWrite  DataStoreName=oTilt  DataStoreElements=oTilt.oIsr_.oState_.fUbPostlpf_  IndexOptions=Index vector (dialog)  Indices=1  OutputSizes=1
  Data Store Write16 : DataStoreWrite  DataStoreName=oTilt  DataStoreElements=oTilt.oIsr_.oState_.fUcPostlpf_  IndexOptions=Index vector (dialog)  Indices=1  OutputSizes=1
  Data Store Write19 : DataStoreWrite  DataStoreName=oTilt  DataStoreElements=oTilt.oIsr_.oState_.fUdcPostlpf_  IndexOptions=Index vector (dialog)  Indices=1  OutputSizes=1
  Data Store Write2 : DataStoreWrite  DataStoreName=oTilt  DataStoreElements=oTilt.oIsr_.oIn_.oAdcData_.fIc_  IndexOptions=Index vector (dialog)  Indices=1  OutputSizes=1
  Data Store Write3 : DataStoreWrite  DataStoreName=oTilt  DataStoreElements=oTilt.oIsr_.oIn_.oAdcData_.fIdc_  IndexOptions=Index vector (dialog)  Indices=1  OutputSizes=1
  Data Store Write4 : DataStoreWrite  DataStoreName=oTilt  DataStoreElements=oTilt.oIsr_.oIn_.oAdcData_.fUa_  IndexOptions=Index vector (dialog)  Indices=1  OutputSizes=1
  Data Store Write5 : DataStoreWrite  DataStoreName=oTilt  DataStoreElements=oTilt.oIsr_.oIn_.oAdcData_.fUb_  IndexOptions=Index vector (dialog)  Indices=1  OutputSizes=1
  Data Store Write6 : DataStoreWrite  DataStoreName=oTilt  DataStoreElements=oTilt.oIsr_.oIn_.oAdcData_.fUc_  IndexOptions=Index vector (dialog)  Indices=1  OutputSizes=1
  Data Store Write7 : DataStoreWrite  DataStoreName=oTilt  DataStoreElements=oTilt.oIsr_.oIn_.oAdcData_.fUdc_  IndexOptions=Index vector (dialog)  Indices=1  OutputSizes=1
  Data Store Write8 : DataStoreWrite  DataStoreName=oTilt  DataStoreElements=oTilt.oIsr_.oIn_.oAdcData_.fAuxiliaryEncoderFloat_  IndexOptions=Index vector (dialog)  Indices=1  OutputSizes=1
  Data Store Write9 : DataStoreWrite  DataStoreName=oTilt  DataStoreElements=oTilt.oIsr_.oIn_.oAdcData_.fMotorEncoderFloat_  IndexOptions=Index vector (dialog)  Indices=1  OutputSizes=1
  wires:
  Bus Selector/7 -> Data Store Write6/1, Data Store Write16/1  "<fUc_>"
  Bus Selector/10 -> Data Store Write9/1  "<fMotorEncoderFloat_>"
  Bus Selector/8 -> Data Store Write19/1, Data Store Write13/1, Data Store Write7/1  "<fUdc_>"
  Bus Selector/4 -> Data Store Write3/1  "<fIdc_>"
  Bus Selector/2 -> Data Store Write1/1  "<fIb_>"
  TiltMotorAdcFeedback/1 -> Bus Selector/1
  Bus Selector/11 -> Data Store Write10/1  "<fMotorSensorSpeed_>"
  Bus Selector/1 -> Data Store Write/1  "<fIa_>"
  Bus Selector/6 -> Data Store Write5/1, Data Store Write15/1  "<fUb_>"
  Bus Selector/3 -> Data Store Write2/1  "<fIc_>"
  Bus Selector/5 -> Data Store Write4/1, Data Store Write14/1  "<fUa_>"
  Bus Selector/12 -> Data Store Write11/1  "<fOutputEncoderFloat_>"
  Bus Selector/13 -> Data Store Write12/1  "<fOutputSensorSpeed_>"
  Bus Selector/9 -> Data Store Write8/1  "<fAuxiliaryEncoderFloat_>"

== system Target_Control_System/Target_Control_System/InterruptFunction/pitchMotor_dataToMain/Variant Subsystem ==
  note: 1) Add Subsystem or Model blocks as valid variant choices.
      | 2) You cannot connect blocks at this level. At simulation, connectivity is automatically
      | determined, based on the active variant and port name matching.
  Subsystem1 : Subsystem  VariantControl=(default)
  VP_leader_follower_postion_copy : Subsystem  VariantControl=TARGET_CODE_GEN==1

== system Target_Control_System/Target_Control_System/InterruptFunction/pitchMotor_isrSchedule/Triggered Subsystem ==
  Trigger : TriggerPort  VariantControl=Variant
  Function-Call Generator : simulink/Ports & Subsystems/Function-Call Generator  sample_time=-1  numberOfIterations=1  DisallowWideOutput=off
  Output : Outport
  wires:
  Function-Call Generator/1 -> Output/1
